simulink model "CEngDsT_VD"  (R2016b)
settings: configuration reference "CodeGenConfigSet" (kept outside this file)
values from neighbouring files (symbols this model uses):
  CEngDsT_facSerPT1_C = Calibration.Parameter    [init_CEngDsT_VD.m]    (also in init_CEngDsT_VD_SIL.m = Simulink.Parameter)
  CEngDsT_RmpSlpNeg_C = Calibration.Parameter    [init_CEngDsT_VD.m]    (also in init_CEngDsT_VD_SIL.m = Simulink.Parameter)
  CEngDsT_RmpSlpPos_C = Calibration.Parameter    [init_CEngDsT_VD.m]    (also in init_CEngDsT_VD_SIL.m = Simulink.Parameter)
  CEngDsT_tDflCold_C = Calibration.Parameter    [init_CEngDsT_VD.m]    (also in init_CEngDsT_VD_SIL.m = Simulink.Parameter)
  CEngDsT_tDflWarm_C = Calibration.Parameter    [init_CEngDsT_VD.m]    (also in init_CEngDsT_VD_SIL.m = Simulink.Parameter)
  SigTst_swtCEngDsT_C = Calibration.Parameter    [init_CEngDsT_VD.m]    (also in init_CEngDsT_VD_SIL.m = Simulink.Parameter)
  SigTst_tCEngDsT_C = Calibration.Parameter    [init_CEngDsT_VD.m]    (also in init_CEngDsT_VD_SIL.m = Simulink.Parameter)
undefined symbols (not defined in the file or in its folder): CEngDst_switch_conv, CEngDsT_VD_DT, EngState_conv, Switch_conv
libraries: CXLib x8
settings Model: Creator=Administrator  LastModifiedBy=dulinggang
settings ConfigSetRef: SourceLocation=Base Workspace

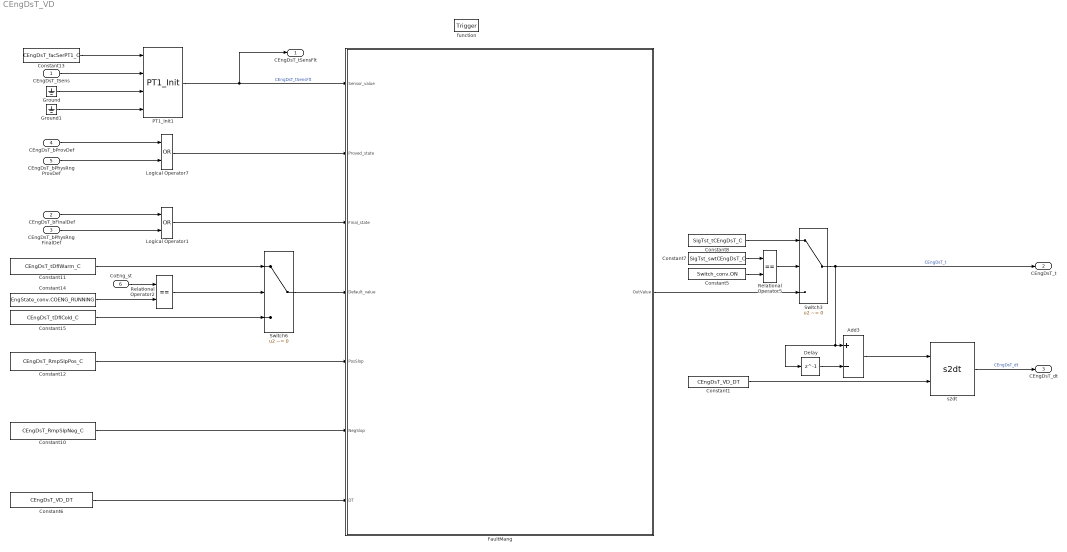
== system CEngDsT_VD ==
  CEngDsT_tSens : Inport  Tag=deg  Description=Sensed engine coolant temperature  OutMin=-200  OutMax=200  OutDataTypeStr=Temp_deg
  CEngDsT_bFinalDef : Inport  Description=Status Sensor of the coolant temperature finally defect  Port=2  OutMin=0  OutMax=1  OutDataTypeStr=boolean
  CEngDsT_bPhysRngFinalDef : Inport  Description=Status Sensor of the CEngDsT physical Signal range check finally defect  Port=3  OutMin=0  OutMax=1  OutDataTypeStr=boolean
  CEngDsT_bProvDef : Inport  Description=Status Sensor of the coolant temperature temporary defect  Port=4  OutMin=0  OutMax=1  OutDataTypeStr=boolean
  CEngDsT_bPhysRngProvDef : Inport  Description=Status Sensor of the CEngDsT physical Signal range check temporary defect  Port=5  OutMin=0  OutMax=1  OutDataTypeStr=boolean
  CoEng_st : Inport  Description=Engine coordinator state  Port=6  OutDataTypeStr=Enum: EngState_conv
  function : TriggerPort  TriggerType=function-call  VariantControl=Variant
  Add3 : Sum  Inputs=+-  OutDataTypeStr=Inherit: Inherit via back propagation  InputSameDT=on
  Constant1 : Constant  Value=CEngDsT_VD_DT  SampleTime=-1
  Constant10 : Constant  Value=CEngDsT_RmpSlpNeg_C  SampleTime=-1
  Constant11 : Constant  Value=CEngDsT_tDflWarm_C  SampleTime=-1
  Constant12 : Constant  Value=CEngDsT_RmpSlpPos_C  SampleTime=-1
  Constant13 : Constant  Value=CEngDsT_facSerPT1_C  SampleTime=-1
  Constant14 : Constant  Value=EngState_conv.COENG_RUNNING  OutDataTypeStr=Inherit: Inherit via back propagation
  Constant15 : Constant  Value=CEngDsT_tDflCold_C  SampleTime=-1
  Constant5 : Constant  Value=Switch_conv.ON  OutDataTypeStr=Inherit: Inherit via back propagation
  Constant6 : Constant  Value=CEngDsT_VD_DT  SampleTime=-1
  Constant7 : Constant  Value=SigTst_swtCEngDsT_C  SampleTime=-1
  Constant8 : Constant  Value=SigTst_tCEngDsT_C  SampleTime=-1
  Delay : Delay  DialogController=Simulink.DDGSource  DelayLength=1  InitialCondition=0
  FaultMang : Subsystem
  Ground : Ground
  Ground1 : Ground
  Logical Operator1 : Logic  Operator=OR  OutDataTypeStr=boolean
  Logical Operator7 : Logic  Operator=OR  OutDataTypeStr=boolean
  PT1_Init1 : CXLib/PT1_Init
  Relational Operator2 : RelationalOperator  Operator===  OutDataTypeStr=boolean  RndMeth=Nearest  InputSameDT=on
  Relational Operator5 : RelationalOperator  Operator===  OutDataTypeStr=boolean  RndMeth=Simplest  InputSameDT=on
  Switch3 : Switch  Criteria=u2 ~= 0  Threshold=CEngDst_switch_conv.OFF  InputSameDT=on
  Switch6 : Switch  Criteria=u2 ~= 0  InputSameDT=on
  s2dt : CXLib/s2dt
  CEngDsT_tSensFlt : Outport  Tag=deg  Description=engine coolant sensor temperature without speed up  OutMin=-200  OutMax=200  OutDataTypeStr=Temp_deg
  CEngDsT_t : Outport  Tag=deg  Description=engine coolant temperature after filter  Port=2  OutMin=-200  OutMax=200  OutDataTypeStr=Temp_deg
  CEngDsT_dt : Outport  Tag=deg/s  Description=temperature change rate  Port=3  OutMin=-200  OutMax=200  OutDataTypeStr=Temp_deg_s
  wires:
  Delay/1 -> Add3/2
  Switch3/1 -> Delay/1, Add3/1, CEngDsT_t/1  "CEngDsT_t"
  CoEng_st/1 -> Relational Operator2/1
  Relational Operator2/1 -> Switch6/2
  Constant11/1 -> Switch6/1
  Constant15/1 -> Switch6/3
  Constant8/1 -> Switch3/1
  Constant13/1 -> PT1_Init1/1
  Constant14/1 -> Relational Operator2/2
  s2dt/1 -> CEngDsT_dt/1  "CEngDsT_dt"
  Relational Operator5/1 -> Switch3/2
  Constant7/1 -> Relational Operator5/1
  Constant5/1 -> Relational Operator5/2
  Add3/1 -> s2dt/1
  Constant1/1 -> s2dt/2
  CEngDsT_tSens/1 -> PT1_Init1/2
  Logical Operator7/1 -> FaultMang/2(Proved_state)
  CEngDsT_bProvDef/1 -> Logical Operator7/1
  CEngDsT_bPhysRngProvDef/1 -> Logical Operator7/2
  Logical Operator1/1 -> FaultMang/3(Final_state)
  CEngDsT_bPhysRngFinalDef/1 -> Logical Operator1/2
  CEngDsT_bFinalDef/1 -> Logical Operator1/1
  PT1_Init1/1 -> CEngDsT_tSensFlt/1, FaultMang/1(Sensor_value)  "CEngDsT_tSensFlt"
  Switch6/1 -> FaultMang/4(Default_value)
  Constant12/1 -> FaultMang/5(PosSlop)
  Constant10/1 -> FaultMang/6(NegSlop)
  FaultMang/1(OutValue) -> Switch3/3
  Ground/1 -> PT1_Init1/3
  Constant6/1 -> FaultMang/7(DT)
  Ground1/1 -> PT1_Init1/4

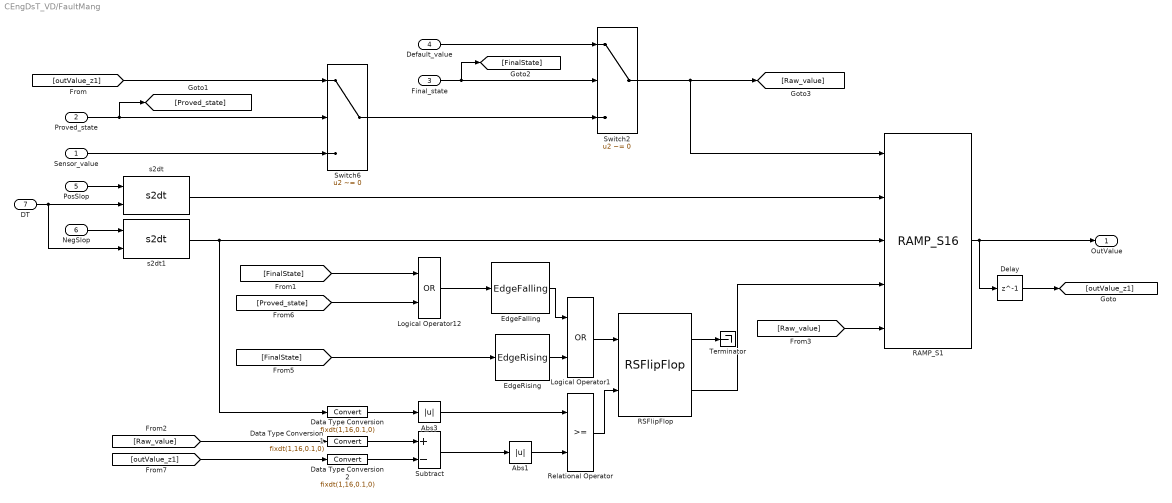
== system CEngDsT_VD/FaultMang ==
  Sensor_value : Inport
  Proved_state : Inport  Port=2
  Final_state : Inport  Port=3
  Default_value : Inport  Port=4
  PosSlop : Inport  Port=5
  NegSlop : Inport  Port=6
  DT : Inport  Port=7
  Abs1 : Abs  OutDataTypeStr=Inherit: Inherit via back propagation
  Abs3 : Abs  OutDataTypeStr=Inherit: Inherit via back propagation
  Data Type Conversion : DataTypeConversion  OutDataTypeStr=fixdt(1,16,0.1,0)  SaturateOnIntegerOverflow=on
  Data Type Conversion1 : DataTypeConversion  OutDataTypeStr=fixdt(1,16,0.1,0)
  Data Type Conversion2 : DataTypeConversion  OutDataTypeStr=fixdt(1,16,0.1,0)
  Delay : Delay  DialogController=Simulink.DDGSource  DelayLength=1  InitialCondition=0
  EdgeFalling : CXLib/EdgeFalling
  EdgeRising : CXLib/EdgeRising
  Logical Operator1 : Logic  Operator=OR  OutDataTypeStr=boolean
  Logical Operator12 : Logic  Operator=OR  OutDataTypeStr=boolean
  RAMP_S1 : CXLib/RAMP_S16
  RSFlipFlop : CXLib/RSFlipFlop
  Relational Operator : RelationalOperator  OutDataTypeStr=boolean  RndMeth=Simplest
  Subtract : Sum  Inputs=+-  OutDataTypeStr=Inherit: Inherit via back propagation  SaturateOnIntegerOverflow=on
  Switch2 : Switch  Criteria=u2 ~= 0  InputSameDT=on
  Switch6 : Switch  Criteria=u2 ~= 0  InputSameDT=on
  Terminator : Terminator
  s2dt : CXLib/s2dt
  s2dt1 : CXLib/s2dt
  OutValue : Outport
  wires:
  Switch2/1 -> RAMP_S1/1, [Raw_value]
  Logical Operator12/1 -> EdgeFalling/1
  s2dt/1 -> RAMP_S1/2
  RSFlipFlop/1 -> Terminator/1
  Relational Operator/1 -> RSFlipFlop/2
  PosSlop/1 -> s2dt/1
  NegSlop/1 -> s2dt1/1
  RAMP_S1/1 -> OutValue/1, Delay/1
  Default_value/1 -> Switch2/1
  Switch6/1 -> Switch2/3
  Delay/1 -> [outValue_z1]
  [outValue_z1] -> Switch6/1
  Final_state/1 -> [FinalState], Switch2/2
  DT/1 -> s2dt1/2, s2dt/2
  [FinalState] -> Logical Operator12/1
  Proved_state/1 -> Switch6/2, [Proved_state]
  [FinalState] -> EdgeRising/1
  [Proved_state] -> Logical Operator12/2
  Sensor_value/1 -> Switch6/3
  s2dt1/1 -> Data Type Conversion/1, RAMP_S1/3
  [Raw_value] -> Data Type Conversion1/1
  [outValue_z1] -> Data Type Conversion2/1
  Abs3/1 -> Relational Operator/1
  Data Type Conversion/1 -> Abs3/1
  [Raw_value] -> RAMP_S1/5
  Data Type Conversion1/1 -> Subtract/1
  Data Type Conversion2/1 -> Subtract/2
  Subtract/1 -> Abs1/1
  Abs1/1 -> Relational Operator/2
  Logical Operator1/1 -> RSFlipFlop/1
  EdgeRising/1 -> Logical Operator1/2
  EdgeFalling/1 -> Logical Operator1/1
  RSFlipFlop/2 -> RAMP_S1/4
